simulink model "Greedy_Advance_L"  (R2015a)
settings: Solver=ode3  StartTime=0.0  StopTime=300  FixedStep=0.01  MaxStep=0.01  RelTol=1e-3
values from neighbouring files (symbols this model uses):
  Imax = 1000    [Gradient_Descent_Greedy_3rd.m]
  n0 = Periodic_Solution(time_shift(j)*100+1,4)    [Gradient_Descent_Greedy_3rd.m]
  Periodic_Solution = Periodic_Solution(101:end,:)    [Gradient_Descent_Greedy_3rd.m]    (also in Periodic_Solution_JFK_1000lux.mat = [0 0.00999999999999 0.02 0.03 0.04 0.05 0.0599999999999 0.06)
  Tol = 0.05    [Gradient_Descent_Greedy_3rd.m]
  x0 = Periodic_Solution(time_shift(j)*100+1,2)    [Gradient_Descent_Greedy_3rd.m]
  xc0 = Periodic_Solution(time_shift(j)*100+1,3)    [Gradient_Descent_Greedy_3rd.m]
undefined symbols (not defined in the file or in its folder): f
settings Model: Creator=wangf7  LastModifiedBy=Jiawei Yin
settings OptimizationCC: ExpressionDepthLimit=2147483647
settings DebuggingCC: UnderspecifiedInitializationDetection=Classic  MergeDetectMultiDrivingBlocksExec=none  SolverPrmCheckMsg=warning  StateNameClashWarn=warning

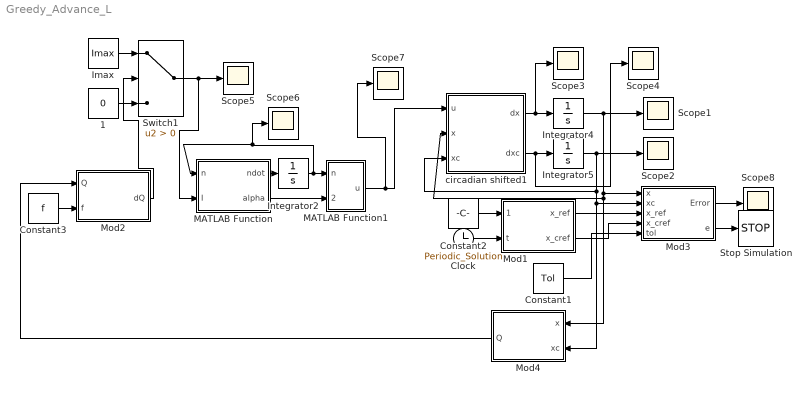
== system Greedy_Advance_L ==
  1 : Constant  Value=0
  Clock : Clock
  Constant1 : Constant  Value=Tol
  Constant2 : Constant  Value=Periodic_Solution
  Constant3 : Constant  Value=f
  Imax : Constant  Value=Imax
  Integrator2 : Integrator  InitialCondition=n0
  Integrator4 : Integrator  InitialCondition=x0
  Integrator5 : Integrator  InitialCondition=xc0
  MATLAB Function : MATLAB Function  TreatAsAtomicUnit=on
      settings: PermitHierarchicalResolution=ParametersOnly
  MATLAB Function1 : MATLAB Function  TreatAsAtomicUnit=on
      settings: PermitHierarchicalResolution=ParametersOnly
  Mod1 : MATLAB Function  TreatAsAtomicUnit=on
      settings: PermitHierarchicalResolution=ParametersOnly
  Mod2 : MATLAB Function  TreatAsAtomicUnit=on
      settings: PermitHierarchicalResolution=ParametersOnly
  Mod3 : MATLAB Function  TreatAsAtomicUnit=on
      settings: PermitHierarchicalResolution=ParametersOnly
  Mod4 : MATLAB Function  TreatAsAtomicUnit=on
      settings: PermitHierarchicalResolution=ParametersOnly
  Scope{1..8} (8 alike) : Scope
      Scope1 settings: TimeRange=auto  MaxDataPoints=50000000  SaveName=x  YMin=-0.9968  YMax=-0.7968  SampleTime=-1  DataFormat=Array
      Scope2 settings: TimeRange=auto  MaxDataPoints=50000000  SaveName=xc  YMin=0.38292  YMax=0.58292  SampleTime=-1  DataFormat=Array
      Scope3 settings: TimeRange=auto  MaxDataPoints=50000000  SaveName=dx  YMin=0.56158  YMax=0.76158  SampleTime=-1  DataFormat=Array
      Scope4 settings: TimeRange=auto  MaxDataPoints=50000000  SaveName=dxc  YMin=0.52134  YMax=0.72134  SampleTime=-1  DataFormat=Array
      Scope5 settings: TimeRange=auto  MaxDataPoints=50000000  SaveName=I  YMin=9000.00000  YMax=11000.00000  SampleTime=-1  DataFormat=Array
      Scope6 settings: TimeRange=auto  MaxDataPoints=50000000000  SaveName=n  YMin=0.0074  YMax=0.0274  SampleTime=-1  DataFormat=Array
      Scope7 settings: TimeRange=auto  MaxDataPoints=50000000  SaveName=u  YMin=0.43727  YMax=0.63727  SampleTime=-1  DataFormat=Array
      Scope8 settings: TimeRange=auto  MaxDataPoints=50000000  SaveName=Error  YMin=0.06416  YMax=0.08416  SampleTime=-1  DataFormat=Array
  Stop Simulation : Stop
  Switch1 : Switch  Criteria=u2 > Threshold
  circadian shifted1 : MATLAB Function  TreatAsAtomicUnit=on
      settings: PermitHierarchicalResolution=ParametersOnly
  wires:
  Imax/1 -> Switch1/1
  1/1 -> Switch1/3
  Constant3/1 -> Mod2/2(f)
  Switch1/1 -> MATLAB Function/2(I), Scope5/1
  circadian shifted1/1(dx) -> Scope3/1, Integrator4/1
  circadian shifted1/2(dxc) -> Scope4/1, Integrator5/1
  Integrator4/1 -> Scope1/1, Mod3/1(x), Mod4/1(x), circadian shifted1/2(x)
  Integrator5/1 -> Scope2/1, Mod4/2(xc), Mod3/2(xc), circadian shifted1/3(xc)
  Mod2/1(dQ) -> Switch1/2
  Mod3/2(e) -> Stop Simulation/1
  Constant2/1 -> Mod1/1(Periodic_Solution)
  Clock/1 -> Mod1/2(t)
  Mod1/1(x_ref) -> Mod3/3(x_ref)
  Mod1/2(x_cref) -> Mod3/4(x_cref)
  Constant1/1 -> Mod3/5(tol)
  Mod4/1(Q) -> Mod2/1(Q)
  MATLAB Function/1(ndot) -> Integrator2/1
  Integrator2/1 -> MATLAB Function/1(n), Scope6/1, MATLAB Function1/1(n)
  MATLAB Function/2(alpha) -> MATLAB Function1/2(alpha)
  MATLAB Function1/1(u) -> Scope7/1, circadian shifted1/1(u)
  Mod3/1(Error) -> Scope8/1

== matlab function Greedy_Advance_L/Mod3 ==
  data: Error output; x input; xc input; e output; x_ref input; x_cref input; tol input
function [Error,e] = fcn(x,xc,x_ref,x_cref,tol)
%#codegen
Error=(x-x_ref)^2+(xc-x_cref)^2;
e=Error<tol;

== matlab function Greedy_Advance_L/Mod1 ==
  data: Periodic_Solution input; x_ref output; t input; x_cref output
function [x_ref,x_cref] = fcn(Periodic_Solution,t)
%#codegen
x_ref=interp1q(Periodic_Solution(:,1),Periodic_Solution(:,2),t);
x_cref=interp1q(Periodic_Solution(:,1),Periodic_Solution(:,3),t);

== matlab function Greedy_Advance_L/circadian shifted1 ==
  data: u input; dx output; x input; xc input; dxc output
function [dx,dxc] = fcn(u,x,xc)

k=0.55;
mu=0.13;
q=1/3;
B=(1-0.4*x)*(1-0.4*xc)*u;
tau=24.2;

dx = pi*(xc+mu*(x/3+4*x^3/3-256*x^7/105)+B)/12;
dxc = pi*(q*B*xc-x*((24/0.99729/tau)^2+k*B))/12;
% dR1 = -pi*R1*(mu*(1/3+4*x^2-256*x^6/15)-0.4*(1-0.4*xc)*u)/12-pi*R2*(-0.4*q*(1-0.4*xc)*xc*u-(24/0.99729/tau)^2-k*(1-0.8*x)*(1-0.4*xc)*u)/12;
% dR2 = -pi*R1*(1-0.4*(1-0.4*x)*u)/12-pi*R2*(q*(1-0.4*x)*(1-0.8*xc)*u+0.4*k*x*(1-0.4*x)*u)/12;

== matlab function Greedy_Advance_L/Mod2 ==
  data: Q input; dQ output; f input
function dQ = fcn(Q,f)
%#codegen

dQ=interp1q(f(:,1),f(:,2),Q);

== matlab function Greedy_Advance_L/Mod4 ==
  data: x input; Q output; xc input
function Q = fcn(x,xc)
%#codegen

Q=mod(atan2(-xc,x),2*pi);

== matlab function Greedy_Advance_L/MATLAB Function ==
  data: n input; I input; ndot output; alpha output
function [ndot,alpha] = fcn(n,I)

alpha0=0.05;
beta=0.0075;
I0=9500;
alpha=alpha0*(I/I0)^0.5;
ndot=60*[alpha*(1-n)-beta*n];

== matlab function Greedy_Advance_L/MATLAB Function1 ==
  data: n input; u output; alpha input
function u = fcn(n,alpha)
%#codegen
u=33.75*alpha*(1-n);
